simulink model "Read_Encoder"  (R2024b)
settings: Solver=FixedStepAuto  StartTime=0.0  StopTime=20  FixedStep=0.01  RelTol=1e-3  EnableMultiTasking=on
libraries: stm32g4xxblockslib x4, stm32f4xxblockslib x2, simulink x1
settings Model: STM32="{\"AnalogInput\":{\"ID\":\"BasicKit:1\"},\"DigitalPortWrite\":{\"ID\":\"BasicKit:3\"},\"DigitalPortRead\":[{\"ID\":\"BasicKit:5\"},{\"ID\":\"BasicKit:7\"},{\"ID\":\"BasicKit:13\"},{\"ID\":\"BasicKit:14\"},{\"ID\":\"QEI:40\"},{\"ID\":\"QEI:41\"},{\"ID\":\"Read_Encoder:40\"},{\"ID\":\"Read_Encoder:41\"}],\"EncoderBlockForG4\":[{\"ID\":\"BasicKit:9\"},{\"ID\":\"QEI:60\"},{\"ID\":\"QEI:61\"},{\"ID\":\"QEI:62\"},{\"ID\":\"Read_Encoder:62\"},{\"ID\":\"Read_Encoder:61\"},{\"ID\":\"Read_Encoder:60\"}],\"HardwareInterrupt\":{\"ID\":\"Read_Encoder:142\"}}"  ExtModeBatchMode=on  Creator=beamk  LastModifiedBy=pboon
settings OptimizationCC: DefaultParameterBehavior=Inlined  EnhancedBackFolding=on  PassReuseOutputArgsAs=Individual arguments  ZeroExternalMemoryAtStartup=off  ZeroInternalMemoryAtStartup=off  MaxStackSize=512  OptimizeBlockOrder=speed  DifferentSizesBufferReuse=on  OptimizationCustomize=off  EfficientTunableParamExpr=on
settings DebuggingCC: ParameterTunabilityLossMsg=error
settings HardwareCC: ProdBitPerPointer=32  ProdBitPerSizeT=32  ProdBitPerPtrDiffT=32  ProdLargestAtomicInteger=Long  ProdLargestAtomicFloat=Double  ProdWordSize=32  ProdLongLongMode=on  ProdHWDeviceType=ARM Compatible->ARM Cortex-M
settings SFSimCC: MATLABDynamicMemAlloc=off
settings RTWCC: Description=Embedded Coder  SystemTargetFile=ert.tlc  HardwareBoard=STM32G4xx Based  TemplateMakefile=ert_default_tmf  Toolchain=GNU Tools for ARM Embedded Processors
settings CodeAppCC: ForceParamTrailComments=on  IgnoreCustomStorageClasses=off  OperatorAnnotations=on  SimulinkDataObjDesc=on  SFDataObjDesc=on  InsertBlockDesc=on
settings ERTTargetCC: TargetLangStandard=C99 (ISO)  CodeReplacementLibrary=ARM Cortex-M  SupportContinuousTime=on  ExtModeTransport=3  ExtModeStaticAlloc=on  ExtModeStaticAllocSize=2048  ExtModeMexFile=ext_xcp  ExtModeIntrfLevel=Level2 - Open

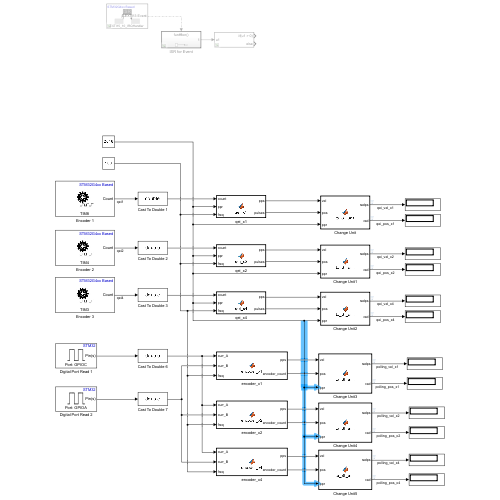
[thumbnail: Simulink's stored preview of the top-level diagram]
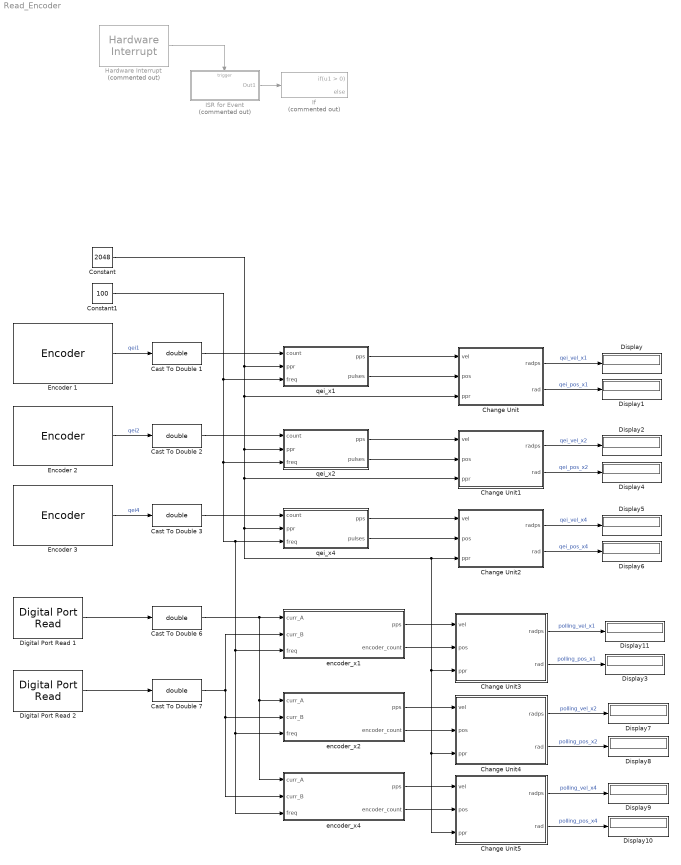
== system Read_Encoder ==
  Cast To Double {1..3,6..7} (5 alike) : DataTypeConversion  OutDataTypeStr=double  SaturateOnIntegerOverflow=off  RndMeth=Floor
  Change Unit : MATLAB Function  TreatAsAtomicUnit=on
  Change Unit1 : MATLAB Function  TreatAsAtomicUnit=on
  Change Unit2 : MATLAB Function  TreatAsAtomicUnit=on
  Change Unit3 : MATLAB Function  TreatAsAtomicUnit=on
  Change Unit4 : MATLAB Function  TreatAsAtomicUnit=on
  Change Unit5 : MATLAB Function  TreatAsAtomicUnit=on
  Constant : Constant  Value=2048
  Constant1 : Constant  Value=100
  Digital Port Read 1 : stm32f4xxblockslib/Digital Port Read  PortName=GPIOC  PinNumber=[7]  ReadOperation=on  IOAsArray=on  SampleTime=-1  EnableSimPort=off  hoistedMaskSrc=ECSoC/ECSimCodegen/Digital Port Read
      settings: LibrarySourceBlock=stm32g4xxblockslib/Digital Port Read
  Digital Port Read 2 : stm32f4xxblockslib/Digital Port Read  PortName=GPIOA  PinNumber=[9]  ReadOperation=on  IOAsArray=on  SampleTime=-1  EnableSimPort=off  hoistedMaskSrc=ECSoC/ECSimCodegen/Digital Port Read
      settings: LibrarySourceBlock=stm32g4xxblockslib/Digital Port Read
  Display{,1..11} (12 alike) : Display
  Encoder 1 : stm32g4xxblockslib/Encoder  TimerModule=TIM8  EnableResetInput=off  OutputCountAfterFirstIndex=off  OutputValidIndex=off  OutputDirection=off  OutputStatus=off  SampleTime=-1
  Encoder 2 : stm32g4xxblockslib/Encoder  TimerModule=TIM4  EnableResetInput=off  OutputCountAfterFirstIndex=off  OutputValidIndex=off  OutputDirection=off  OutputStatus=off  SampleTime=-1
  Encoder 3 : stm32g4xxblockslib/Encoder  TimerModule=TIM3  EnableResetInput=off  OutputCountAfterFirstIndex=off  OutputValidIndex=off  OutputDirection=off  OutputStatus=off  SampleTime=-1
  Hardware Interrupt : stm32g4xxblockslib/Hardware Interrupt  Commented=on  ISRGroup=External interrupts (EXTI)  ISRName=EXTI15_10_IRQHandler  ISRNumber=55  EventsList={ 'off', 'EXTI15 Event', '1'; 'off', 'EXTI14 Event', '2'; 'on', 'EXTI13 Event', '3'; 'off', 'EXTI12 Event', '4'; 'off', 'EXTI11 Event', '5'; 'off', 'EXTI10 Event', '6'; 'off', 'Custom event', '7' }  SelectedEvents={'EXTI13 Event'}  TaskPriority=30  DisablePreemption=off  ClearInterruptFlagsAtEndOfEvent=off  InterruptDefinitionFile=$(TARGET_ROOT)/registry/interrupts/STM32F4xxBased_interrupts.xml  HardwareBoard=STM32G4xx Based  EnableSimPort=off
  ISR for Event : Subsystem  Commented=on  TreatAsAtomicUnit=on
  If : If  Commented=on
  encoder_x1 : MATLAB Function  TreatAsAtomicUnit=on
  encoder_x2 : MATLAB Function  TreatAsAtomicUnit=on
  encoder_x4 : MATLAB Function  TreatAsAtomicUnit=on
  qei_x1 : MATLAB Function  TreatAsAtomicUnit=on
  qei_x2 : MATLAB Function  TreatAsAtomicUnit=on
  qei_x4 : MATLAB Function  TreatAsAtomicUnit=on
  wires:
  Cast To Double 2/1 -> qei_x2/1(count)
  Cast To Double 1/1 -> qei_x1/1(count)
  Cast To Double 3/1 -> qei_x4/1(count)
  Digital Port Read 1/1 -> Cast To Double 6/1
  Encoder 1/1 -> Cast To Double 1/1  "qei1"
  Encoder 2/1 -> Cast To Double 2/1  "qei2"
  Encoder 3/1 -> Cast To Double 3/1  "qei4"
  Constant/1 -> Change Unit/3(ppr), Change Unit1/3(ppr), Change Unit5/3(ppr), Change Unit4/3(ppr), Change Unit3/3(ppr), Change Unit2/3(ppr), qei_x4/2(ppr), qei_x2/2(ppr), qei_x1/2(ppr)
  Constant1/1 -> encoder_x4/3(freq), encoder_x2/3(freq), encoder_x1/3(freq), qei_x4/3(freq), qei_x2/3(freq), qei_x1/3(freq)
  qei_x1/1(pps) -> Change Unit/1(vel)
  qei_x1/2(pulses) -> Change Unit/2(pos)
  qei_x2/1(pps) -> Change Unit1/1(vel)
  qei_x2/2(pulses) -> Change Unit1/2(pos)
  qei_x4/1(pps) -> Change Unit2/1(vel)
  qei_x4/2(pulses) -> Change Unit2/2(pos)
  Change Unit2/1(radps) -> Display5/1  "qei_vel_x4"
  Change Unit2/2(rad) -> Display6/1  "qei_pos_x4"
  Change Unit1/2(rad) -> Display4/1  "qei_pos_x2"
  Change Unit1/1(radps) -> Display2/1  "qei_vel_x2"
  Change Unit/2(rad) -> Display1/1  "qei_pos_x1"
  Change Unit/1(radps) -> Display/1  "qei_vel_x1"
  Digital Port Read 2/1 -> Cast To Double 7/1
  Cast To Double 6/1 -> encoder_x4/1(curr_A), encoder_x2/1(curr_A), encoder_x1/1(curr_A)
  Cast To Double 7/1 -> encoder_x2/2(curr_B), encoder_x4/2(curr_B), encoder_x1/2(curr_B)
  Change Unit4/1(radps) -> Display7/1  "polling_vel_x2"
  Change Unit3/2(rad) -> Display3/1  "polling_pos_x1"
  Change Unit4/2(rad) -> Display8/1  "polling_pos_x2"
  Change Unit5/2(rad) -> Display10/1  "polling_pos_x4"
  Change Unit5/1(radps) -> Display9/1  "polling_vel_x4"
  Change Unit3/1(radps) -> Display11/1  "polling_vel_x1"
  encoder_x2/1(pps) -> Change Unit4/1(vel)
  encoder_x2/2(encoder_count) -> Change Unit4/2(pos)
  encoder_x4/1(pps) -> Change Unit5/1(vel)
  encoder_x4/2(encoder_count) -> Change Unit5/2(pos)
  Hardware Interrupt/1 -> ISR for Event/Trigger
  ISR for Event/1(Out1) -> If/1
  encoder_x1/1(pps) -> Change Unit3/1(vel)
  encoder_x1/2(encoder_count) -> Change Unit3/2(pos)

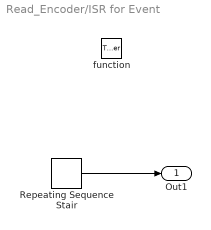
== system Read_Encoder/ISR for Event ==
  function : TriggerPort  TriggerType=function-call  VariantControl=(inherit)
  Repeating Sequence Stair : simulink/Sources/Repeating Sequence Stair  OutValues=[1 0]  tsamp=-1  OutMin=[]  OutMax=[]  OutDataTypeStr=double  OutputDataTypeScalingMode=double  OutDataType=fixdt(0,8)  ConRadixGroup=Best Precision: Vector-wise  OutScaling=2^-12
  Out1 : Outport
  wires:
  Repeating Sequence Stair/1 -> Out1/1

== matlab function Read_Encoder/Change Unit3 ==
  data: vel input; radps output; pos input; rad output; ppr input
function [radps, rad] = to_SI_unit(vel, pos, ppr)
    radps = (vel * 2 * pi) / ppr;

    rad = (pos * 2 * pi) / ppr;
end

== matlab function Read_Encoder/Change Unit4 ==
  data: vel input; radps output; pos input; rad output; ppr input
function [radps, rad] = to_SI_unit(vel, pos, ppr)
    radps = (vel * 2 * pi) / ppr;

    rad = (pos * 2 * pi) / ppr;
end

== matlab function Read_Encoder/Change Unit5 ==
  data: vel input; radps output; pos input; rad output; ppr input
function [radps, rad] = to_SI_unit(vel, pos, ppr)
    radps = (vel * 2 * pi) / ppr;

    rad = (pos * 2 * pi) / ppr;
end

== matlab function Read_Encoder/qei_x2 ==
  data: count input; pps output; pulses output; ppr input; freq input
function [pps, pulses] = qei_x2(count, ppr, freq)
enc_period = 65536 - mod(65536,ppr*2);
persistent prev_count
persistent pulses_accum
persistent diff_count

if isempty(prev_count)
    prev_count = 0;
end

if isempty(pulses_accum)
    pulses_accum = 0;
end

if isempty(diff_count)
    diff_count = 0;
end

diff_count = count - prev_count;

if diff_count > enc_period / 2
    diff_count = diff_count - enc_period;
elseif diff_count < -enc_period / 2
    diff_count = diff_count + enc_period;
end

pulses_accum = pulses_accum + diff_count;

pulses = pulses_accum;
pps = double(diff_count)*freq;

prev_count = count;
end

== matlab function Read_Encoder/qei_x4 ==
  data: count input; pps output; pulses output; ppr input; freq input
function [pps, pulses] = qei_x4(count, ppr, freq)
enc_period = 65536 - mod(65536,ppr*4);
persistent prev_count
persistent pulses_accum
persistent diff_count

if isempty(prev_count)
    prev_count = 0;
end

if isempty(pulses_accum)
    pulses_accum = 0;
end

if isempty(diff_count)
    diff_count = 0;
end

diff_count = count - prev_count;

if diff_count > enc_period / 2
    diff_count = diff_count - enc_period;
elseif diff_count < -enc_period / 2
    diff_count = diff_count + enc_period;
end

pulses_accum = pulses_accum + diff_count;

pulses = pulses_accum;
pps = double(diff_count)*freq;

prev_count = count;
end

== matlab function Read_Encoder/Change Unit ==
  data: vel input; radps output; pos input; rad output; ppr input
function [radps, rad] = to_SI_unit(vel, pos, ppr)
    radps = (vel * 2 * pi) / ppr;

    rad = (pos * 2 * pi) / ppr;
end

== matlab function Read_Encoder/encoder_x1 ==
  data: pps output; curr_A input; encoder_count output; curr_B input; freq input
function [pps, encoder_count] =  encoder_x1( curr_A, curr_B, freq)
persistent prev_A
persistent prev_B
persistent count
persistent prev_count

if isempty(prev_A)
    prev_A = 0;
end

if isempty(prev_B)
    prev_B = 0;
end

if isempty(count)
    count = 0;
end

if isempty(prev_count)
    prev_count = 0;
end

if (prev_A == 0) && (curr_A == 1)
    if curr_B == 0
        count = count + 1;
    else
        count = count - 1;
    end
end

encoder_count = count;

diff_count = count - prev_count;

pps = double(diff_count)*freq;

prev_A = curr_A;
prev_B = curr_B;

prev_count = count;
end

== matlab function Read_Encoder/encoder_x2 ==
  data: pps output; curr_A input; encoder_count output; curr_B input; freq input
function [pps, encoder_count]= encoder_x2(curr_A, curr_B, freq)
persistent prev_A
persistent prev_B
persistent count
persistent prev_count

if isempty(prev_A)
    prev_A = 0;
end

if isempty(prev_B)
    prev_B = 0;
end

if isempty(count)
    count = 0;
end

if isempty(prev_count)
    prev_count = 0;
end

if curr_A ~= prev_A
    if (prev_A == curr_B)
        count = count + 1;
    else
        count = count - 1;
    end
end

encoder_count = count;

diff_count = count - prev_count;

pps = double(diff_count)*freq;

prev_A = curr_A;
prev_B = curr_B;

prev_count = count;
end

== matlab function Read_Encoder/encoder_x4 ==
  data: pps output; curr_A input; encoder_count output; curr_B input; freq input
function [pps, encoder_count]= encoder_x4(curr_A, curr_B, freq)
persistent prev_A
persistent prev_B
persistent count
persistent prev_count

if isempty(prev_A)
    prev_A = 0;
end

if isempty(prev_B)
    prev_B = 0;
end

if isempty(count)
    count = 0;
end

if isempty(prev_count)
    prev_count = 0;
end

if curr_A ~= prev_A  
    if curr_A ~= curr_B
        count = count + 1;  
    else
        count = count - 1;  
    end
end

if curr_B ~= prev_B  
    if curr_A == curr_B
        count = count + 1; 
    else
        count = count - 1; 
    end
end

encoder_count = count;

diff_count = count - prev_count;

pps = double(diff_count)*freq;

prev_A = curr_A;
prev_B = curr_B;

prev_count = count;
end

== matlab function Read_Encoder/Change Unit1 ==
  data: vel input; radps output; pos input; rad output; ppr input
function [radps, rad] = to_SI_unit(vel, pos, ppr)
    radps = (vel * 2 * pi) / ppr;

    rad = (pos * 2 * pi) / ppr;
end

== matlab function Read_Encoder/Change Unit2 ==
  data: vel input; radps output; pos input; rad output; ppr input
function [radps, rad] = to_SI_unit(vel, pos, ppr)
    radps = (vel * 2 * pi) / ppr;

    rad = (pos * 2 * pi) / ppr;
end

== matlab function Read_Encoder/qei_x1 ==
  data: count input; pps output; pulses output; ppr input; freq input
function [pps, pulses] = qei_x1(count, ppr, freq)
enc_period = 65536 - mod(65536,ppr);
persistent prev_count
persistent pulses_accum
persistent diff_count    

if isempty(prev_count)
    prev_count = 0;
end

if isempty(pulses_accum)
    pulses_accum = 0;
end

if isempty(diff_count)
    diff_count = 0;
end

diff_count = count - prev_count;

if diff_count > enc_period / 2
    diff_count = diff_count - enc_period;
elseif diff_count < -enc_period / 2
    diff_count = diff_count + enc_period;
end

pulses_accum = pulses_accum + diff_count;

pulses = pulses_accum;
pps = double(diff_count)*freq;

prev_count = count;
end
